simulink model "SimRLC"  (R2024a)
settings: Solver=VariableStepAuto  StartTime=0.0  StopTime=0.001  RelTol=1e-3
values from neighbouring files (symbols this model uses):
  C = 0.1e-6    (= 1e-07)    [RLC.m]    (also in RLCsimulinkparametros.m)
  L = 6e-3    (= 0.006)    [RLC.m]    (also in RLCsimulinkparametros.m)
  R = 100    [RLC.m]    (also in RLCsimulinkparametros.m)
settings Model: LastModifiedBy=100117273
settings RTWCC: GPUComputeCapability=3.5

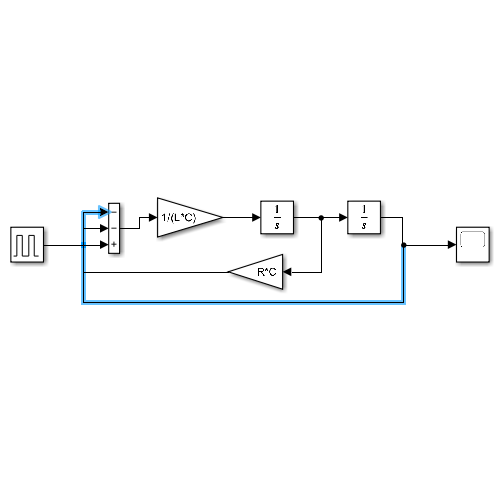
[thumbnail: Simulink's stored preview of the top-level diagram]
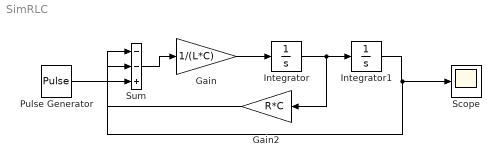
== system SimRLC ==
  Gain : Gain  Gain=1/(L*C)
  Gain2 : Gain  Gain=R*C
  Integrator : Integrator
  Integrator1 : Integrator
  Pulse Generator : DiscretePulseGenerator  PulseType=Time based  Period=0.02  PulseWidth=50
  Scope : Scope
  Sum : Sum  Inputs=--+
  wires:
  Pulse Generator/1 -> Sum/3
  Sum/1 -> Gain/1
  Gain/1 -> Integrator/1
  Integrator/1 -> Gain2/1, Integrator1/1
  Gain2/1 -> Sum/2
  Integrator1/1 -> Sum/1, Scope/1
